simulink library "LIB_Control"  (R2018b)
settings: Solver=VariableStepAuto  StartTime=0.0  StopTime=10.0  RelTol=1e-3
undefined symbols (not defined in the file or in its folder): tControlPeriod
libraries: LIB_AirVolumeProcessing x1, LIB_InputsProcessing x1, LIB_OutputsProcessing x1, LIB_RespiratorSupervisor x1, LIB_UserCommand x1, LIB_Warning x1
settings Model: Creator=BRAUL  LastModifiedBy=BRAUL

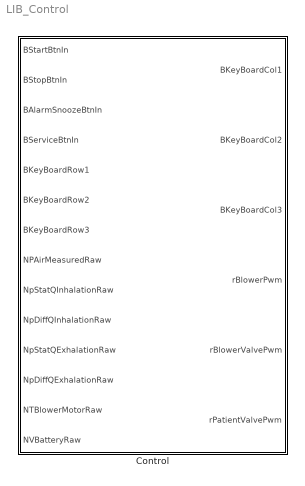
== system LIB_Control ==
  Control : Subsystem  TreatAsAtomicUnit=on  SystemSampleTime=tControlPeriod
      settings: AttributesFormatString=%<ReferenceBlock>

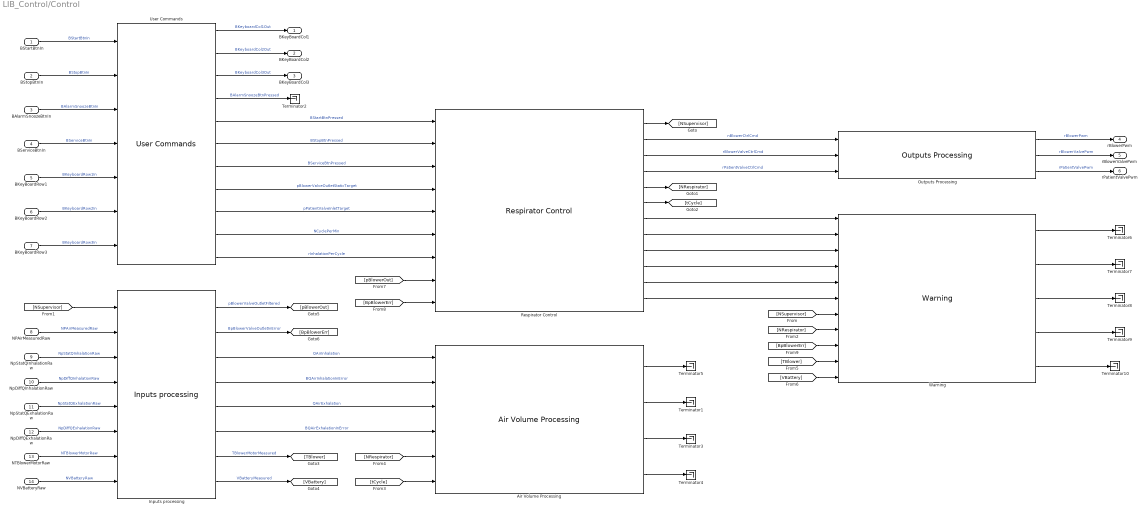
== system LIB_Control/Control ==
  BStartBtnIn : Inport  OutDataTypeStr=boolean
  BStopBtnIn : Inport  Port=2  OutDataTypeStr=boolean
  BAlarmSnoozeBtnIn : Inport  Port=3  OutDataTypeStr=boolean
  BServiceBtnIn : Inport  Port=4  OutDataTypeStr=boolean
  BKeyBoardRow1 : Inport  Port=5  OutDataTypeStr=boolean  PortDimensions=1
  BKeyBoardRow2 : Inport  Port=6  OutDataTypeStr=boolean  PortDimensions=1
  BKeyBoardRow3 : Inport  Port=7  OutDataTypeStr=boolean  PortDimensions=1
  NPAirMeasuredRaw : Inport  Port=8
  NpStatQInhalationRaw : Inport  Port=9  OutDataTypeStr=single
  NpDiffQInhalationRaw : Inport  Port=10  OutDataTypeStr=single
  NpStatQExhalationRaw : Inport  Port=11  OutDataTypeStr=single
  NpDiffQExhalationRaw : Inport  Port=12  OutDataTypeStr=single
  NTBlowerMotorRaw : Inport  Port=13
  NVBatteryRaw : Inport  Port=14
  Air Volume Processing : LIB_AirVolumeProcessing/Air Volume Processing  SystemSampleTime=-1
      settings: AttributesFormatString=%<ReferenceBlock>
  Inputs processing : LIB_InputsProcessing/Inputs processing  SystemSampleTime=-1
      settings: AttributesFormatString=%<ReferenceBlock>
  Outputs Processing : LIB_OutputsProcessing/Outputs Processing  SystemSampleTime=-1
      settings: AttributesFormatString=%<ReferenceBlock>
  Respirator Control : LIB_RespiratorSupervisor/Respirator Control  SystemSampleTime=-1
      settings: AttributesFormatString=%<ReferenceBlock>
  Terminator{1..10} (10 alike) : Terminator
  User Commands : LIB_UserCommand/User Commands  SystemSampleTime=-1
      settings: AttributesFormatString=%<ReferenceBlock>
  Warning : LIB_Warning/Warning  SystemSampleTime=-1
      settings: AttributesFormatString=%<ReferenceBlock>
  BKeyBoardCol1 : Outport  OutDataTypeStr=boolean  PortDimensions=1
  BKeyBoardCol2 : Outport  Port=2  OutDataTypeStr=boolean  PortDimensions=1
  BKeyBoardCol3 : Outport  Port=3  OutDataTypeStr=boolean  PortDimensions=1
  rBlowerPwm : Outport  Port=4
  rBlowerValvePwm : Outport  Port=5
  rPatientValvePwm : Outport  Port=6
  wires:
  Warning/5 -> Terminator10/1
  Warning/4 -> Terminator9/1
  Warning/3 -> Terminator8/1
  Warning/2 -> Terminator7/1
  Warning/1 -> Terminator6/1
  Inputs processing/5 -> Air Volume Processing/3  "QAirExhalation"
  Inputs processing/4 -> Air Volume Processing/2  "BQAirInhalationInError"
  Inputs processing/3 -> Air Volume Processing/1  "QAirInhalation"
  Inputs processing/6 -> Air Volume Processing/4  "BQAirExhalationInError"
  NpDiffQExhalationRaw/1 -> Inputs processing/6  "NpDiffQExhalationRaw"
  NpStatQExhalationRaw/1 -> Inputs processing/5  "NpStatQExhalationRaw"
  NpDiffQInhalationRaw/1 -> Inputs processing/4  "NpDiffQInhalationRaw"
  NpStatQInhalationRaw/1 -> Inputs processing/3  "NpStatQInhalationRaw"
  Inputs processing/2 -> [BpBlowerErr]  "BpBlowerValveOutletInError"
  User Commands/3 -> BKeyBoardCol3/1  "BKeyboardCol3Out"
  User Commands/2 -> BKeyBoardCol2/1  "BKeyboardCol2Out"
  User Commands/1 -> BKeyBoardCol1/1  "BKeyboardCol1Out"
  BKeyBoardRow3/1 -> User Commands/7  "BKeyboardRow3In"
  BKeyBoardRow2/1 -> User Commands/6  "BKeyboardRow2In"
  BKeyBoardRow1/1 -> User Commands/5  "BKeyboardRow1In"
  Inputs processing/8 -> [VBattery]  "VBatteryMeasured"
  Inputs processing/7 -> [TBlower]  "TBlowerMotorMeasured"
  NVBatteryRaw/1 -> Inputs processing/8  "NVBatteryRaw"
  NTBlowerMotorRaw/1 -> Inputs processing/7  "NTBlowerMotorRaw"
  User Commands/7 -> Respirator Control/3  "BServiceBtnPressed"
  User Commands/4 -> Terminator2/1  "BAlarmSnoozeBtnPressed"
  User Commands/6 -> Respirator Control/2  "BStopBtnPressed"
  User Commands/5 -> Respirator Control/1  "BStartBtnPressed"
  BServiceBtnIn/1 -> User Commands/4  "BServiceBtnIn"
  BAlarmSnoozeBtnIn/1 -> User Commands/3  "BAlarmSnoozeBtnIn"
  BStopBtnIn/1 -> User Commands/2  "BStopBtnIn"
  BStartBtnIn/1 -> User Commands/1  "BStartBtnIn"
  Respirator Control/4 -> Outputs Processing/3  "rPatientValveCtrlCmd"
  Respirator Control/3 -> Outputs Processing/2  "rBlowerValveCtrlCmd"
  Respirator Control/2 -> Outputs Processing/1  "nBlowerCtrlCmd"
  Outputs Processing/3 -> rPatientValvePwm/1  "rPatientValvePwm"
  Outputs Processing/1 -> rBlowerPwm/1  "rBlowerPwm"
  Inputs processing/1 -> [pBlowerOut]  "pBlowerValveOutletFiltered"
  User Commands/11 -> Respirator Control/7  "rInhalationPerCycle"
  Outputs Processing/2 -> rBlowerValvePwm/1  "rBlowerValvePwm"
  NPAirMeasuredRaw/1 -> Inputs processing/2  "NPAirMeasuredRaw"
  User Commands/8 -> Respirator Control/4  "pBlowerValveOutletStaticTarget"
  User Commands/9 -> Respirator Control/5  "pPatientValveInletTarget"
  User Commands/10 -> Respirator Control/6  "NCyclePerMin"
  Respirator Control/7 -> Warning/1
  Respirator Control/8 -> Warning/2
  Respirator Control/9 -> Warning/3
  Respirator Control/10 -> Warning/4
  Respirator Control/11 -> Warning/5
  Respirator Control/12 -> Warning/6
  Respirator Control/1 -> [NSupervisor]
  [NSupervisor] -> Warning/7
  [NSupervisor] -> Inputs processing/1
  Respirator Control/5 -> [NRespirator]
  [NRespirator] -> Warning/8
  Respirator Control/6 -> [tCycle]
  [tCycle] -> Air Volume Processing/6
  [NRespirator] -> Air Volume Processing/5
  [VBattery] -> Warning/11
  [TBlower] -> Warning/10
  [pBlowerOut] -> Respirator Control/8
  [BpBlowerErr] -> Respirator Control/9
  [BpBlowerErr] -> Warning/9
  Air Volume Processing/1 -> Terminator5/1
  Air Volume Processing/2 -> Terminator1/1
  Air Volume Processing/3 -> Terminator3/1
  Air Volume Processing/4 -> Terminator4/1
